simulink model "sm_parts_test_tube_box"  (R2018a)
settings: Solver=VariableStepAuto  StartTime=0.0  StopTime=10.0  RelTol=1e-3  EnableMultiTasking=on
model workspace (MATLAB code in the model file):
  | box_ox = 0.2;
  | box_ix = 0.16;
  | box_oy = 0.32;
  | box_iy = 0.24;
  | box_arc_rad = 0.9;
  | box_arc = 270/2;
  | box_density = 7000;
  | box_color = [0 0.4 0.6];
  | box_color_str = [0.2 0.6 0.2];
  | box_opc = 1;
  | 
  | box_len = 0.3;
undefined symbols (not defined in the file): X, Y, Z
libraries: Multibody_Parts_Lib x16, sm_lib x7, nesl_utility x1
CloseFcn:
  | try,close(h1_sm_parts_test_tube_box),end
  | clear h1_sm_parts_test_tube_box
  | try,close(h2_sm_parts_test_tube_box),end
  | clear h2_sm_parts_test_tube_box
  | try,close(h3_sm_parts_test_tube_box),end
  | clear h3_sm_parts_test_tube_box
  | try,close(h4_sm_parts_test_tube_box),end
  | clear h4_sm_parts_test_tube_box
Description:
  | Box Extrusion Assembly
  | 
  | Copyright 2017-2018 The MathWorks, Inc.
settings Model: Creator=smiller  LastModifiedBy=smiller
settings DataIOCC: LimitDataPoints=on
settings OptimizationCC: LifeSpan=inf
settings DebuggingCC: AllowSymbolicDim=off  SFUnexpectedBacktrackingDiag=warning  SFNoUnconditionalDefaultTransitionDiag=warning  SFExecutionAtInitializationDiag=none
settings CodeAppCC: StateflowObjectComments=on
settings GRTTargetCC: TargetLangStandard=C89/C90 (ANSI)  GeneratePreprocessorConditionals=Disable all
settings ConfigComp: CovMetricSettings=dw  CovHtmlReporting=on  CovSaveCumulativeToWorkspaceVar=on  CovSaveSingleToWorkspaceVar=on  CovExternalEMLEnable=off  CovSFcnEnable=off
settings SimscapeCC: SimscapeNormalizeSystem=off  SimscapeLogType=all  SimscapeLogDataHistory=10000
settings ConfigurationSet: Description=SimMechanics 2G
settings DiagnosticsConfigSet: SimMechanicsUnconnectedFramePorts=none
settings ExplorerConfigSet: InternalSimMechanicsExplorerSettings="<ExplorerConfiguration><canonicalview>planar_xy</canonicalview><AnimationSetting><BasePlaybackSpeed>1.0</BasePlaybackSpeed><PlaybackSpeedFactor>1.0</PlaybackSpeedFactor></AnimationSetting><TilePanel><TileInfo><Tiles Columns=\"2\" Count=\"2\" Rows=\"1\"><Column Left=\"2\" Weight=\"0.4997\"/><Column Left=\"326\" Weight=\"0.5003\"/><Column Left=\"650\"/><Row Top=\"2\" Weight=\"1\"/><Row Top=\"397\"/><Tile Height=\"1\" Width=\"1\" X=\"0\" Y=\"0\"/><Tile Height=\"1\" Width=\"1\" X=\"1\" Y=\"0\"/></Tiles></TileInfo><SceneInfo><SceneViewer><BGColor><R>1</R><G>1</G><B>1</B></BGColor><Camera><DoPerspective>off</DoPerspective><Position><X>-5.9424842451961553</X><Y>3.1544382471445216</Y><Z>1.0231052648354773</Z></Position><Center><X>-1.5674737523807989</X><Y>1.7193917656705162</Y><Z>-2.1787783296558909</Z></Center><Up><X>0.21656061186599329</X><Y>0.96656645249549644</Y><Z>-0.13729819481150571</Z></Up><ViewLimDist>1</ViewLimDist><YLim>2.5038796600229083</YLim><XLim>2.043321484215586</XLim></Camera></SceneViewer><SceneViewer><BGColor><R>1</R><G>1</G><B>1</B></BGColor><Camera><DoPerspective>off</DoPerspective><Position><X>-7.7586025295667289</X><Y>0.15532774559300866</Y><Z>-0.14253475616197075</Z></Position><Center><X>-1.2208320076024302</X><Y>0.15532774559300866</Y><Z>-0.14253475616197075</Z></Center><Up><X>-0</X><Y>1</Y><Z>0</Z></Up><ViewLimDist>1</ViewLimDist><YLim>1.417704930741299</YLim><XLim>1.1569353709417336</XLim></Camera></SceneViewer></SceneInfo></TilePanel><MechEditorPanel><Cameras/><GfxPanelCameraMap/><VideoCreator><PlaybackSpeedRatio>1.0</PlaybackSpeedRatio><FrameRate>30</FrameRate><VideoFormat>Motion JPEG AVI</VideoFormat><FrameSize>auto</FrameSize></VideoCreator></MechEditorPanel></ExplorerConfiguration>"

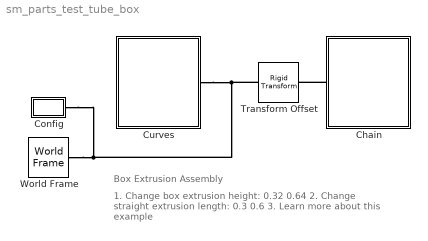
== system sm_parts_test_tube_box ==
  note: Box Extrusion Assembly
  note: 1. Change box extrusion height: 0.32 0.64
      | 2. Change straight extrusion length: 0.3 0.6
      | 3. Learn more about this example
  Chain : Subsystem  Tag=PublishSubsystem
  Config : Subsystem
  Curves : Subsystem  Tag=PublishSubsystem
  Transform Offset : sm_lib/Frames and Transforms/Rigid Transform  TranslationMethod=StandardAxis  TranslationStandardOffset=-2  TranslationLengthUnit=m  TranslationStandardAxis=+Z  TranslationCartesianOffset=[0 0 0]  TranslationROffset=0  TranslationROffsetUnits=m  TranslationZOffset=0  TranslationZOffsetUnits=m  TranslationThetaOffset=0  TranslationThetaOffsetUnits=deg  RotationMethod=None  RotationAngleUnits=deg  RotationStandardAxis=+Z  RotationAngle=0.0  RotationArbitraryAxis=[0 0 1]  FollAlignAxisA=+X  BaseAlignAxisA=+Y  FollAlignAxisB=+Y  BaseAlignAxisB=+Z  RotationSequenceAxes=FollowerAxes  RotationSequence=XYX  RotationSequenceAngles=[0 0 0]  RotationSequenceAnglesUnits=deg  RotationMatrix=[1 0 0; 0 1 0; 0 0 1]
  World Frame : sm_lib/Frames and Transforms/World Frame
  connections:
  Curves/LConn1 -- Config/LConn1 -- World Frame/RConn1 -- Transform Offset/LConn1
  Chain/LConn1 -- Transform Offset/RConn1

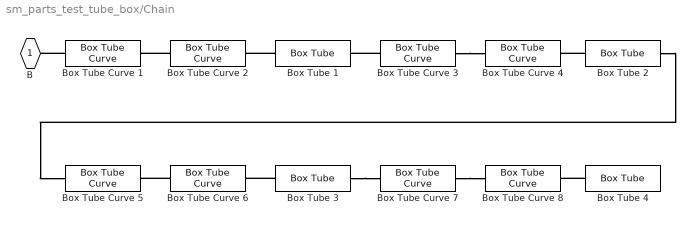
== system sm_parts_test_tube_box/Chain ==
  Box Tube Curve 1 : Multibody_Parts_Lib/Extrusions/Box Tube Curve  box_ox=box_ox  box_ix=box_ix  box_oy=box_oy  box_iy=box_iy  arc_rad=box_arc_rad  arc_angle=box_arc  popup_arcdir=Z  box_rho=box_density  box_color=box_color  box_opc=box_opc
      settings: SourceProductName=Simscape Multibody Parts Library
  Box Tube Curve 3 : Multibody_Parts_Lib/Extrusions/Box Tube Curve  box_ox=box_ox  box_ix=box_ix  box_oy=box_oy  box_iy=box_iy  arc_rad=box_arc_rad  arc_angle=box_arc  popup_arcdir=Y  box_rho=box_density  box_color=box_color  box_opc=box_opc
      settings: SourceProductName=Simscape Multibody Parts Library
  Box Tube Curve 4 : Multibody_Parts_Lib/Extrusions/Box Tube Curve  box_ox=box_ox  box_ix=box_ix  box_oy=box_oy  box_iy=box_iy  arc_rad=box_arc_rad  arc_angle=box_arc  popup_arcdir=Y  box_rho=box_density  box_color=box_color  box_opc=box_opc
      settings: SourceProductName=Simscape Multibody Parts Library
  Box Tube Curve 5 : Multibody_Parts_Lib/Extrusions/Box Tube Curve  box_ox=box_ox  box_ix=box_ix  box_oy=box_oy  box_iy=box_iy  arc_rad=box_arc_rad  arc_angle=-box_arc  popup_arcdir=Z  box_rho=box_density  box_color=box_color  box_opc=box_opc
      settings: SourceProductName=Simscape Multibody Parts Library
  Box Tube Curve 6 : Multibody_Parts_Lib/Extrusions/Box Tube Curve  box_ox=box_ox  box_ix=box_ix  box_oy=box_oy  box_iy=box_iy  arc_rad=box_arc_rad  arc_angle=-box_arc  popup_arcdir=Z  box_rho=box_density  box_color=box_color  box_opc=box_opc
      settings: SourceProductName=Simscape Multibody Parts Library
  Box Tube Curve 7 : Multibody_Parts_Lib/Extrusions/Box Tube Curve  box_ox=box_ox  box_ix=box_ix  box_oy=box_oy  box_iy=box_iy  arc_rad=box_arc_rad  arc_angle=-box_arc  popup_arcdir=Y  box_rho=box_density  box_color=box_color  box_opc=box_opc
      settings: SourceProductName=Simscape Multibody Parts Library
  Box Tube Curve 8 : Multibody_Parts_Lib/Extrusions/Box Tube Curve  box_ox=box_ox  box_ix=box_ix  box_oy=box_oy  box_iy=box_iy  arc_rad=box_arc_rad  arc_angle=-box_arc  popup_arcdir=Y  box_rho=box_density  box_color=box_color  box_opc=box_opc
      settings: SourceProductName=Simscape Multibody Parts Library
  Box Tube Curve 2 : Multibody_Parts_Lib/Extrusions/Box Tube Curve  box_ox=box_ox  box_ix=box_ix  box_oy=box_oy  box_iy=box_iy  arc_rad=box_arc_rad  arc_angle=box_arc  popup_arcdir=Z  box_rho=box_density  box_color=box_color  box_opc=box_opc
      settings: SourceProductName=Simscape Multibody Parts Library
  Box Tube {1..4} (4 alike) : Multibody_Parts_Lib/Extrusions/Box Tube  box_ox=box_ox  box_ix=box_ix  box_oy=box_oy  box_iy=box_iy  box_len=box_len  box_rho=box_density  box_color=box_color_str  box_opc=box_opc
      settings: SourceProductName=Simscape Multibody Parts Library
  B : PMIOPort  Side=Left
  connections:
  Box Tube Curve 1/LConn1 -- B/RConn1
  Box Tube 1/LConn1 -- Box Tube Curve 2/RConn1
  Box Tube Curve 2/LConn1 -- Box Tube Curve 1/RConn1
  Box Tube Curve 3/LConn1 -- Box Tube 1/RConn1
  Box Tube Curve 3/RConn1 -- Box Tube Curve 4/LConn1
  Box Tube 2/LConn1 -- Box Tube Curve 4/RConn1
  Box Tube 4/LConn1 -- Box Tube Curve 8/RConn1
  Box Tube Curve 7/RConn1 -- Box Tube Curve 8/LConn1
  Box Tube 3/RConn1 -- Box Tube Curve 7/LConn1
  Box Tube Curve 6/LConn1 -- Box Tube Curve 5/RConn1
  Box Tube 3/LConn1 -- Box Tube Curve 6/RConn1
  Box Tube 2/RConn1 -- Box Tube Curve 5/LConn1

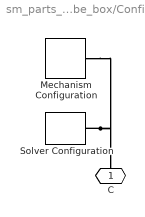
== system sm_parts_test_tube_box/Config ==
  Mechanism Configuration : sm_lib/Utilities/Mechanism Configuration  UniformGravity=Constant  GravityVector=[0 -1 0]*9.80665  GravityUnits=m/s^2  LinearizationDelta=0.001
  Solver Configuration : nesl_utility/Solver Configuration  PhysicalDomain=network_engine_domain  SubClassName=solver  LeftPortType=input  RightPortType=generic  Tones=[]  Harmonics=[]  SimulateNoise=off  Profile=off  UseLocalSampling=off  EnableSwitchedLinearOptims=on  FrequencyDomain=off  UseCCode=off  RelTol=0.001  AbsTol=1e-06  MinStep=1e-09  ToWorkspace=off  RevertToSquareIcSolve=off  NumHomotopyIterations=100  PhasorMode=off  PhasorModeNumHarmonics=1  DoDC=off  ResidualTolerance=1e-09  UseLocalSolver=off  LocalSolverChoice=NE_BACKWARD_EULER_ADVANCER  LocalSolverSampleTime=0.001  DoFixedCost=off  MaxNonlinIter=3  MaxModeIter=2  LinearAlgebra=Sparse  EquationFormulation=NE_TIME_EF  DelaysMemoryBudget=1024  AutomaticFiltering=on  FilteringTimeConstant=0.001
  C : PMIOPort  Side=Left
  connections:
  Solver Configuration/RConn1 -- C/RConn1 -- Mechanism Configuration/RConn1

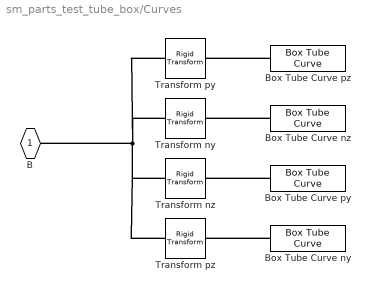
== system sm_parts_test_tube_box/Curves ==
  Box Tube Curve ny : Multibody_Parts_Lib/Extrusions/Box Tube Curve  box_ox=box_ox  box_ix=box_ix  box_oy=box_oy  box_iy=box_iy  arc_rad=box_arc_rad  arc_angle=-60  popup_arcdir=Y  box_rho=box_density  box_color=box_color  box_opc=box_opc
      settings: SourceProductName=Simscape Multibody Parts Library
  Box Tube Curve nz : Multibody_Parts_Lib/Extrusions/Box Tube Curve  box_ox=box_ox  box_ix=box_ix  box_oy=box_oy  box_iy=box_iy  arc_rad=box_arc_rad  arc_angle=-60  popup_arcdir=Z  box_rho=box_density  box_color=box_color  box_opc=box_opc
      settings: SourceProductName=Simscape Multibody Parts Library
  Box Tube Curve py : Multibody_Parts_Lib/Extrusions/Box Tube Curve  box_ox=box_ox  box_ix=box_ix  box_oy=box_oy  box_iy=box_iy  arc_rad=box_arc_rad  arc_angle=60  popup_arcdir=Y  box_rho=box_density  box_color=box_color  box_opc=box_opc
      settings: SourceProductName=Simscape Multibody Parts Library
  Box Tube Curve pz : Multibody_Parts_Lib/Extrusions/Box Tube Curve  box_ox=box_ox  box_ix=box_ix  box_oy=box_oy  box_iy=box_iy  arc_rad=box_arc_rad  arc_angle=60  popup_arcdir=Z  box_rho=box_density  box_color=box_color  box_opc=box_opc
      settings: SourceProductName=Simscape Multibody Parts Library
  Transform ny : sm_lib/Frames and Transforms/Rigid Transform  TranslationMethod=StandardAxis  TranslationStandardOffset=-0.5  TranslationLengthUnit=m  TranslationStandardAxis=+Y  TranslationCartesianOffset=[0 0 0]  TranslationROffset=0  TranslationROffsetUnits=m  TranslationZOffset=0  TranslationZOffsetUnits=m  TranslationThetaOffset=0  TranslationThetaOffsetUnits=deg  RotationMethod=None  RotationAngleUnits=deg  RotationStandardAxis=+Z  RotationAngle=0.0  RotationArbitraryAxis=[0 0 1]  FollAlignAxisA=+X  BaseAlignAxisA=+Y  FollAlignAxisB=+Y  BaseAlignAxisB=+Z  RotationSequenceAxes=FollowerAxes  RotationSequence=XYX  RotationSequenceAngles=[0 0 0]  RotationSequenceAnglesUnits=deg  RotationMatrix=[1 0 0; 0 1 0; 0 0 1]
  Transform nz : sm_lib/Frames and Transforms/Rigid Transform  TranslationMethod=StandardAxis  TranslationStandardOffset=-0.5  TranslationLengthUnit=m  TranslationStandardAxis=+Z  TranslationCartesianOffset=[0 0 0]  TranslationROffset=0  TranslationROffsetUnits=m  TranslationZOffset=0  TranslationZOffsetUnits=m  TranslationThetaOffset=0  TranslationThetaOffsetUnits=deg  RotationMethod=None  RotationAngleUnits=deg  RotationStandardAxis=+Z  RotationAngle=0.0  RotationArbitraryAxis=[0 0 1]  FollAlignAxisA=+X  BaseAlignAxisA=+Y  FollAlignAxisB=+Y  BaseAlignAxisB=+Z  RotationSequenceAxes=FollowerAxes  RotationSequence=XYX  RotationSequenceAngles=[0 0 0]  RotationSequenceAnglesUnits=deg  RotationMatrix=[1 0 0; 0 1 0; 0 0 1]
  Transform py : sm_lib/Frames and Transforms/Rigid Transform  TranslationMethod=StandardAxis  TranslationStandardOffset=0.5  TranslationLengthUnit=m  TranslationStandardAxis=+Y  TranslationCartesianOffset=[0 0 0]  TranslationROffset=0  TranslationROffsetUnits=m  TranslationZOffset=0  TranslationZOffsetUnits=m  TranslationThetaOffset=0  TranslationThetaOffsetUnits=deg  RotationMethod=None  RotationAngleUnits=deg  RotationStandardAxis=+Z  RotationAngle=0.0  RotationArbitraryAxis=[0 0 1]  FollAlignAxisA=+X  BaseAlignAxisA=+Y  FollAlignAxisB=+Y  BaseAlignAxisB=+Z  RotationSequenceAxes=FollowerAxes  RotationSequence=XYX  RotationSequenceAngles=[0 0 0]  RotationSequenceAnglesUnits=deg  RotationMatrix=[1 0 0; 0 1 0; 0 0 1]
  Transform pz : sm_lib/Frames and Transforms/Rigid Transform  TranslationMethod=StandardAxis  TranslationStandardOffset=0.5  TranslationLengthUnit=m  TranslationStandardAxis=+Z  TranslationCartesianOffset=[0 0 0]  TranslationROffset=0  TranslationROffsetUnits=m  TranslationZOffset=0  TranslationZOffsetUnits=m  TranslationThetaOffset=0  TranslationThetaOffsetUnits=deg  RotationMethod=None  RotationAngleUnits=deg  RotationStandardAxis=+Z  RotationAngle=0.0  RotationArbitraryAxis=[0 0 1]  FollAlignAxisA=+X  BaseAlignAxisA=+Y  FollAlignAxisB=+Y  BaseAlignAxisB=+Z  RotationSequenceAxes=FollowerAxes  RotationSequence=XYX  RotationSequenceAngles=[0 0 0]  RotationSequenceAnglesUnits=deg  RotationMatrix=[1 0 0; 0 1 0; 0 0 1]
  B : PMIOPort  Side=Left
  connections:
  Transform pz/LConn1 -- Transform nz/LConn1 -- Transform ny/LConn1 -- Transform py/LConn1 -- B/RConn1
  Box Tube Curve pz/LConn1 -- Transform py/RConn1
  Box Tube Curve nz/LConn1 -- Transform ny/RConn1
  Box Tube Curve py/LConn1 -- Transform nz/RConn1
  Box Tube Curve ny/LConn1 -- Transform pz/RConn1
